simulink model "sampleModel1549"  (R2023a)
settings: Solver=VariableStepAuto  StartTime=0.0  StopTime=10.0  RelTol=1e-3
libraries: hdlsllib x5, simulink x2
settings Model: Creator=user1  LastModifiedBy=user1

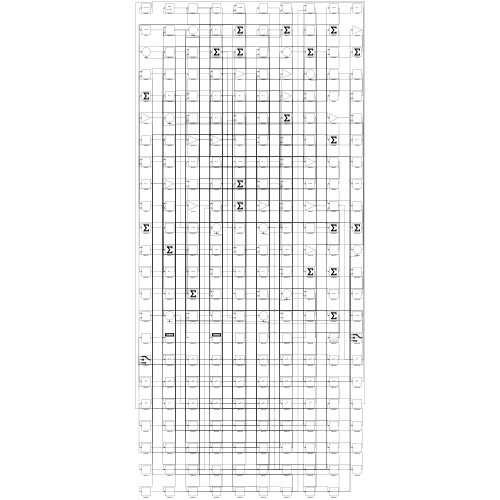
[thumbnail: Simulink's stored preview of the top-level diagram]
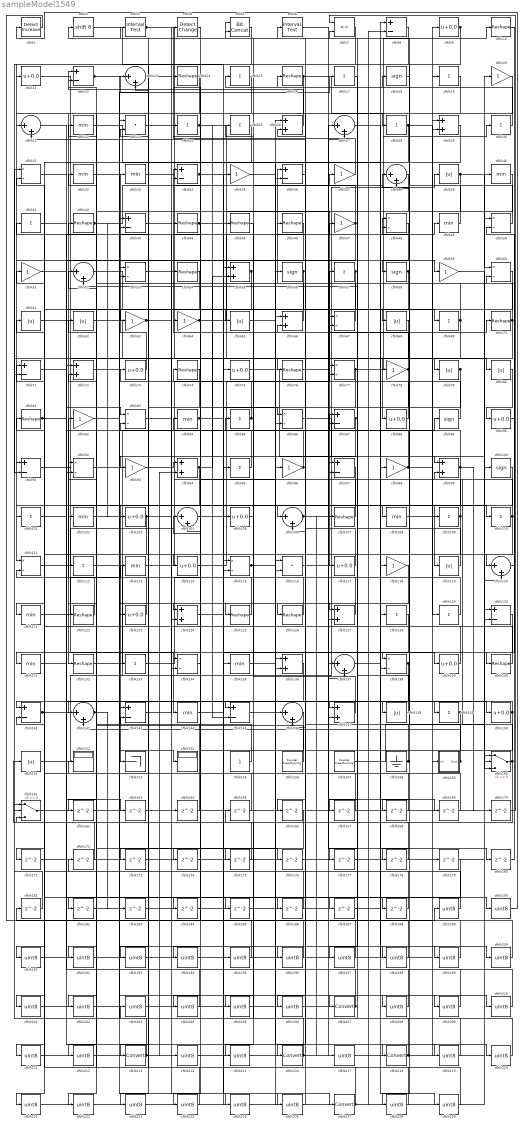
== system sampleModel1549 ==
  cfblk1 : simulink/Logic and Bit Operations/Detect Increase  vinit=0.0  OutDataTypeStr=boolean
      settings: LibrarySourceBlock=|
      | hdlsllib/Logic and Bit
      | Operations/Detect
      | Increase
  cfblk{10,14,16,42,44..46,54,70,74,76,81,107,122,125..126,132,140} (18 alike) : Reshape
  cfblk{18,56,58,89,100} (5 alike) : Signum
  cfblk{15,17,19,24..25,28,30,41,57,69,85,95,101,109..110,112,128..129,133,149} (20 alike) : Sum  Inputs=+
  cfblk{22,32..33,40,49,84,102,108,113,121,131,135,144} (13 alike) : MinMax
  cfblk{9,11,73,75,88,90,103,105,114,117,123,139,150} (13 alike) : Bias  Bias=0.0  SaturateOnIntegerOverflow=off
  cfblk{13,21,27,38,52,104,106,120,137,142,146} (11 alike) : Sum  Inputs=|++
  cfblk{31,48,50,53,60,67,77,83,86,92,111,115,134,138} (14 alike) : Product  Inputs=*/  RndMeth=Zero  SaturateOnIntegerOverflow=on
  cfblk116 : DotProduct  OutDataTypeStr=Inherit: Inherit via internal rule
  cfblk{20,35,37,47,51,59,63..64,78,82,93,96,98,118} (14 alike) : Gain
  cfblk{39,61..62,65,68,79..80,119,148,151} (10 alike) : Abs  SaturateOnIntegerOverflow=off
  cfblk{8,12,34,36,43,71,87,91,97,130,141,143,145} (13 alike) : Sum  Inputs=+-
  cfblk{26,29,55,66,72,94,99,124,127,136,147} (11 alike) : Sum
  cfblk152 : Display
  cfblk153 : Terminator
  cfblk154 : Display
  cfblk155 : Constant  SampleTime=-1
  cfblk156 : hdlsllib/Sources/Counter Free-Running  NumBits=16  tsamp=-1
  cfblk157 : hdlsllib/Sources/Counter Free-Running  NumBits=16  tsamp=-1
  cfblk158 : Ground
  cfblk159 : Subsystem
      settings: LibrarySourceBlock=|
      | hdlsllib/Ports &
      | Subsystems/Subsystem
  cfblk160 : Switch  SaturateOnIntegerOverflow=off  InputSameDT=off
  cfblk161 : Switch  SaturateOnIntegerOverflow=off  InputSameDT=off
  cfblk{162..188} (27 alike) : Delay  SampleTime=1
  cfblk{189..206,208..212,214..215,217,219..226,228..229} (36 alike) : DataTypeConversion  OutDataTypeStr=uint8  SaturateOnIntegerOverflow=off  RndMeth=Floor
  cfblk2 : ArithShift  BitShiftNumber=8
  cfblk{207,213,216,218,227} (5 alike) : DataTypeConversion  SaturateOnIntegerOverflow=off  RndMeth=Floor
  cfblk23 : DotProduct  OutDataTypeStr=Inherit: Inherit via internal rule
  cfblk3 : hdlsllib/Logic and Bit Operations/Interval Test  IntervalClosedRight=on  uplimit=0.5  IntervalClosedLeft=on  lowlimit=-0.5  OutDataTypeStr=boolean
  cfblk4 : simulink/Logic and Bit Operations/Detect Change  vinit=0  OutDataTypeStr=boolean
      settings: LibrarySourceBlock=|
      | hdlsllib/Logic and Bit
      | Operations/Detect
      | Change
  cfblk5 : hdlsllib/Logic and Bit Operations/Bit Concat  numInputs=2
  cfblk6 : hdlsllib/Logic and Bit Operations/Interval Test  IntervalClosedRight=on  uplimit=0.5  IntervalClosedLeft=on  lowlimit=-0.5  OutDataTypeStr=boolean
  cfblk7 : RelationalOperator  Operator=<=  OutDataTypeStr=boolean  InputSameDT=off
  wires:
  cfblk14/1 -> cfblk111/1
  cfblk149/1 -> cfblk206/1, cfblk228/1
  cfblk80/1 -> cfblk90/1
  cfblk73/1 -> cfblk33/1
  cfblk133/1 -> cfblk74/1
  cfblk112/1 -> cfblk39/1
  cfblk141/1 -> cfblk148/1, cfblk87/2
  cfblk9/1 -> cfblk21/1, cfblk38/2
  cfblk46/1 -> cfblk91/1
  cfblk23/1 -> cfblk135/1
  cfblk15/1 -> cfblk132/1
  cfblk34/1 -> cfblk79/1, cfblk145/2
  cfblk77/1 -> cfblk10/1, cfblk123/1
  cfblk84/1 -> cfblk194/1, cfblk226/1
  cfblk45/1 -> cfblk125/1
  cfblk67/1 -> cfblk36/1
  cfblk72/1 -> cfblk207/1
  cfblk155/1 -> cfblk41/1
  cfblk50/1 -> cfblk18/1
  cfblk53/1 -> cfblk100/1
  cfblk61/1 -> cfblk144/1
  cfblk4/1 -> cfblk124/1
  cfblk143/1 -> cfblk48/1
  cfblk113/1 -> cfblk45/1
  cfblk81/1 -> cfblk83/1, cfblk163/1
  cfblk40/1 -> cfblk126/1
  cfblk48/1 -> cfblk58/1
  cfblk122/1 -> cfblk82/1
  cfblk24/1 -> cfblk117/1, cfblk105/1
  cfblk54/1 -> cfblk121/1
  cfblk29/1 -> cfblk213/1
  cfblk110/1 -> cfblk141/1, cfblk48/2
  cfblk22/1 -> cfblk96/1
  cfblk139/1 -> cfblk71/1
  cfblk18/1 -> cfblk108/1
  cfblk132/1 -> cfblk84/1
  cfblk114/1 -> cfblk57/1
  cfblk16/1 -> cfblk28/1, cfblk114/1
  cfblk124/1 -> cfblk138/1
  cfblk33/1 -> cfblk88/1
  cfblk131/1 -> cfblk87/1
  cfblk11/1 -> cfblk80/1
  cfblk58/1 -> cfblk92/2, cfblk168/1
  cfblk127/1 -> cfblk102/1
  cfblk2/1 -> cfblk95/1
  cfblk27/1 -> cfblk98/1
  cfblk94/1 -> cfblk153/1, cfblk55/2, cfblk134/2
  cfblk10/1 -> cfblk140/1
  cfblk158/1 -> cfblk67/1, cfblk21/2
  cfblk148/1 -> cfblk52/2
  cfblk69/1 -> cfblk16/1, cfblk71/2
  cfblk42/1 -> cfblk30/1, cfblk103/1
  cfblk26/1 -> cfblk12/1
  cfblk123/1 -> cfblk51/1
  cfblk78/1 -> cfblk34/1, cfblk127/1
  cfblk3/1 -> cfblk128/1, cfblk109/1
  cfblk157/1 -> cfblk40/1
  cfblk70/1 -> cfblk53/2, cfblk192/1
  cfblk85/1 -> cfblk64/1, cfblk23/2
  cfblk59/1 -> cfblk160/2
  cfblk62/1 -> cfblk78/1
  cfblk125/1 -> cfblk92/1
  cfblk93/1 -> cfblk94/1
  cfblk36/1 -> cfblk106/1
  cfblk63/1 -> cfblk69/1, cfblk208/1
  cfblk98/1 -> cfblk19/1, cfblk44/1
  cfblk31/1 -> cfblk218/1
  cfblk28/1 -> cfblk129/1, cfblk86/2
  cfblk7/1 -> cfblk63/1
  cfblk119/1 -> cfblk67/2
  cfblk49/1 -> cfblk2/1
  cfblk90/1 -> cfblk120/1
  cfblk140/1 -> cfblk54/1
  cfblk156/1 -> cfblk32/1
  cfblk115/1 -> cfblk26/1, cfblk139/1
  cfblk121/1 -> cfblk113/1
  cfblk64/1 -> cfblk9/1, cfblk196/1
  cfblk109/1 -> cfblk147/2, cfblk101/1, cfblk85/1, cfblk178/1
  cfblk96/1 -> cfblk93/1, cfblk83/2
  cfblk8/1 -> cfblk11/1
  cfblk101/1 -> cfblk150/1
  cfblk106/1 -> cfblk110/1, cfblk217/1
  cfblk138/1 -> cfblk166/1, cfblk167/1
  cfblk151/1 -> cfblk35/1
  cfblk52/1 -> cfblk65/1
  cfblk111/1 -> cfblk56/1
  cfblk56/1 -> cfblk171/1, cfblk215/1
  cfblk37/1 -> cfblk4/1
  cfblk71/1 -> cfblk49/1
  cfblk161/1 -> cfblk27/1
  cfblk99/1 -> cfblk73/1, cfblk170/1, cfblk212/1
  cfblk160/1 -> cfblk151/1, cfblk99/2
  cfblk44/1 -> cfblk115/1, cfblk86/1
  cfblk159/1(Out1) -> cfblk38/1, cfblk142/2
  cfblk108/1 -> cfblk119/1
  cfblk89/1 -> cfblk53/1
  cfblk12/1 -> cfblk149/1, cfblk225/1
  cfblk126/1 -> cfblk5/1
  cfblk92/1 -> cfblk154/1
  cfblk86/1 -> cfblk99/1
  cfblk95/1 -> cfblk3/1
  cfblk120/1 -> cfblk50/2
  cfblk91/1 -> cfblk138/2
  cfblk107/1 -> cfblk24/1
  cfblk88/1 -> cfblk14/1
  cfblk103/1 -> cfblk89/1, cfblk202/1
  cfblk150/1 -> cfblk142/1, cfblk145/1, cfblk186/1
  cfblk142/1 -> cfblk182/1, cfblk183/1
  cfblk87/1 -> cfblk124/2, cfblk7/2
  cfblk75/1 -> cfblk160/3
  cfblk116/1 -> cfblk70/1
  cfblk100/1 -> cfblk112/1
  cfblk47/1 -> cfblk25/1, cfblk184/1, cfblk185/1
  cfblk147/1 -> cfblk15/1
  cfblk39/1 -> cfblk60/1, cfblk197/1
  cfblk60/1 -> cfblk76/1
  cfblk57/1 -> cfblk107/1, cfblk127/2
  cfblk51/1 -> cfblk68/1
  cfblk129/1 -> cfblk6/1
  cfblk55/1 -> cfblk133/1, cfblk134/1
  cfblk17/1 -> cfblk147/1
  cfblk20/1 -> cfblk216/1
  cfblk135/1 -> cfblk37/1
  cfblk117/1 -> cfblk66/2
  cfblk13/1 -> cfblk227/1
  cfblk41/1 -> cfblk59/1
  cfblk5/1 -> cfblk91/2
  cfblk145/1 -> cfblk47/1
  cfblk66/1 -> cfblk22/1
  cfblk30/1 -> cfblk5/2
  cfblk68/1 -> cfblk131/1
  cfblk32/1 -> cfblk17/1
  cfblk38/1 -> cfblk122/1
  cfblk79/1 -> cfblk205/1, cfblk223/1
  cfblk19/1 -> cfblk162/1
  cfblk163/1 -> cfblk160/1
  cfblk83/1 -> cfblk164/1
  cfblk164/1 -> cfblk12/2
  cfblk165/1 -> cfblk141/2
  cfblk167/1 -> cfblk26/2
  cfblk168/1 -> cfblk52/1
  cfblk6/1 -> cfblk169/1
  cfblk169/1 -> cfblk77/1
  cfblk170/1 -> cfblk7/1
  cfblk171/1 -> cfblk50/1
  cfblk172/1 -> cfblk111/2
  cfblk74/1 -> cfblk173/1
  cfblk134/1 -> cfblk174/1
  cfblk105/1 -> cfblk175/1
  cfblk175/1 -> cfblk161/2
  cfblk102/1 -> cfblk176/1
  cfblk176/1 -> cfblk120/2
  cfblk128/1 -> cfblk177/1
  cfblk177/1 -> cfblk8/1
  cfblk178/1 -> cfblk106/2
  cfblk76/1 -> cfblk180/1
  cfblk180/1 -> cfblk60/2
  cfblk181/1 -> cfblk161/1
  cfblk182/1 -> cfblk36/2
  cfblk183/1 -> cfblk27/2
  cfblk184/1 -> cfblk115/2
  cfblk186/1 -> cfblk34/2
  cfblk21/1 -> cfblk187/1
  cfblk144/1 -> cfblk188/1
  cfblk188/1 -> cfblk61/1
  cfblk1/1 -> cfblk189/1
  cfblk189/1 -> cfblk62/1
  cfblk174/1 -> cfblk190/1
  cfblk190/1 -> cfblk1/1
  cfblk179/1 -> cfblk191/1
  cfblk191/1 -> cfblk116/2
  cfblk192/1 -> cfblk179/1
  cfblk118/1 -> cfblk193/1
  cfblk193/1 -> cfblk116/1
  cfblk194/1 -> cfblk118/1
  cfblk104/1 -> cfblk195/1
  cfblk195/1 -> cfblk181/1
  cfblk196/1 -> cfblk104/1
  cfblk197/1 -> cfblk104/2
  cfblk43/1 -> cfblk198/1
  cfblk198/1 -> cfblk161/3
  cfblk35/1 -> cfblk199/1
  cfblk199/1 -> cfblk43/1
  cfblk162/1 -> cfblk200/1
  cfblk200/1 -> cfblk43/2
  cfblk136/1 -> cfblk201/1
  cfblk201/1 -> cfblk66/1
  cfblk202/1 -> cfblk136/1
  cfblk203/1 -> cfblk136/2
  cfblk97/1 -> cfblk204/1
  cfblk204/1 -> cfblk42/1
  cfblk205/1 -> cfblk97/1
  cfblk206/1 -> cfblk97/2
  cfblk207/1 -> cfblk143/2, cfblk46/1
  cfblk208/1 -> cfblk72/1
  cfblk82/1 -> cfblk209/1
  cfblk209/1 -> cfblk72/2
  cfblk137/1 -> cfblk210/1
  cfblk210/1 -> cfblk23/1
  cfblk25/1 -> cfblk211/1
  cfblk211/1 -> cfblk137/1
  cfblk212/1 -> cfblk137/2
  cfblk213/1 -> cfblk172/1, cfblk94/2
  cfblk173/1 -> cfblk214/1
  cfblk214/1 -> cfblk29/1
  cfblk215/1 -> cfblk29/2
  cfblk216/1 -> cfblk203/1, cfblk159/1(In1), cfblk143/1
  cfblk217/1 -> cfblk20/1
  cfblk218/1 -> cfblk165/1, cfblk77/2
  cfblk65/1 -> cfblk219/1
  cfblk219/1 -> cfblk31/1
  cfblk185/1 -> cfblk220/1
  cfblk220/1 -> cfblk31/2
  cfblk130/1 -> cfblk221/1
  cfblk221/1 -> cfblk75/1
  cfblk166/1 -> cfblk222/1
  cfblk222/1 -> cfblk130/1
  cfblk223/1 -> cfblk130/2
  cfblk146/1 -> cfblk224/1
  cfblk224/1 -> cfblk81/1
  cfblk225/1 -> cfblk146/1
  cfblk226/1 -> cfblk146/2
  cfblk227/1 -> cfblk55/1, cfblk8/2, cfblk152/1
  cfblk228/1 -> cfblk13/1
  cfblk187/1 -> cfblk229/1
  cfblk229/1 -> cfblk13/2

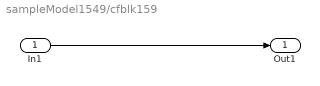
== system sampleModel1549/cfblk159 ==
  In1 : Inport
  Out1 : Outport
  wires:
  In1/1 -> Out1/1
